simulink model "digi_modu2"  (R2019b)
settings: Solver=VariableStepAuto  StartTime=0.0  StopTime=2  RelTol=1e-3
libraries: dsparch4 x1
settings Model: Creator=yango  LastModifiedBy=yango

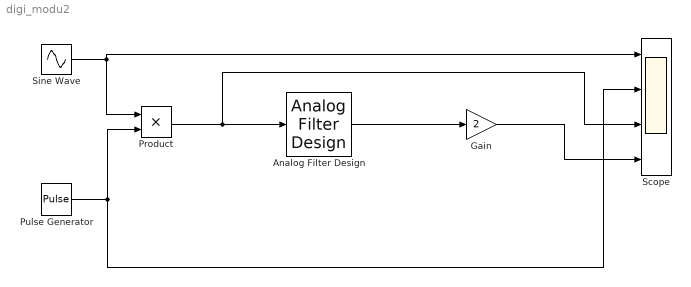
== system digi_modu2 ==
  Analog Filter Design : dsparch4/Analog Filter Design  method=Butterworth  filttype=Lowpass  N=8  Wlo=24*pi  Whi=80  Rp=2  Rs=40
  Gain : Gain  Gain=2
  Product : Product
  Pulse Generator : DiscretePulseGenerator  PulseType=Time based  Period=1/40  PulseWidth=10
  Scope : Scope  NumInputPorts=4
  Sine Wave : Sin  Frequency=20*pi  SampleTime=0
  wires:
  Sine Wave/1 -> Product/1, Scope/1
  Pulse Generator/1 -> Scope/2, Product/2
  Product/1 -> Scope/3, Analog Filter Design/1
  Analog Filter Design/1 -> Gain/1
  Gain/1 -> Scope/4
